simulink model "Cruise_Control"  (R2020b)
settings: Solver=VariableStepAuto  StartTime=0.0  StopTime=10.0  RelTol=1e-3
model workspace (MAT data in the model file):
  b = Simulink.Parameter
  b.Value = 50
  b.DataType = 'auto'
  b.Dimensions = [1 1]
  m1 = Simulink.Parameter
  m1.Value = 1000
  m1.DataType = 'auto'
  m1.Dimensions = [1 1]
settings Model: DataDictionary=Prob3_2005160.sldd  OrderedModelArguments=off  Creator=shoun  LastModifiedBy=shoun

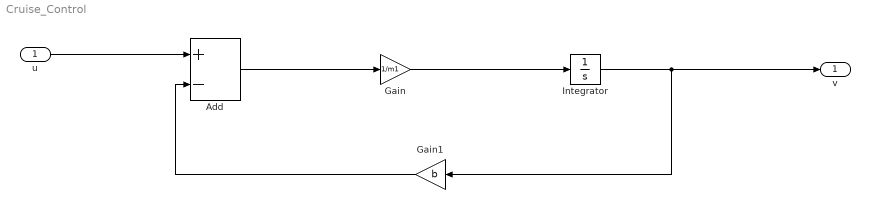
== system Cruise_Control ==
  u : Inport
  Add : Sum  Inputs=+-
  Gain : Gain  Gain=1/m1
  Gain1 : Gain  Gain=b
  Integrator : Integrator
  v : Outport
  wires:
  u/1 -> Add/1
  Add/1 -> Gain/1
  Gain/1 -> Integrator/1
  Integrator/1 -> Gain1/1, v/1
  Gain1/1 -> Add/2
